simulink model "dspmrf_nbpf"  (Simulink 5.0)
settings: Solver=FixedStepDiscrete  SolverMode=SingleTasking  StartTime=0.0  StopTime=inf  RelTol=1e-3  AbsTol=1e-6
PreLoadFcn:
  | load dspmrf_coeffs
libraries: dspmlti3 x4, dspsrcs4 x2, dspsnks4 x2, dspmrf_lib x1
settings Model: Creator=don  LastModifiedBy=schim  ExtModeTrigMode=oneshot  ExtModeArmWhenConnect=off  SaveTime=off  SaveOutput=off  LimitDataPoints=off  IntegerOverflowMsg=none  BlockReductionOpt=off  BooleanDataType=off  RTWOptions=-aRollThreshold=2

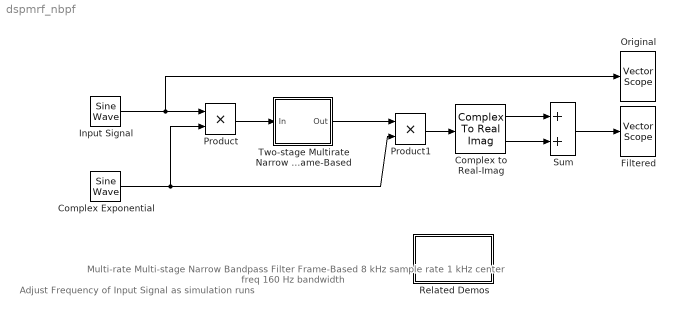
== system dspmrf_nbpf ==
  note: Multi-rate Multi-stage
      | Narrow Bandpass Filter
      | Frame-Based
      |
      | 8 kHz sample rate
      | 1 kHz center freq
      | 160 Hz bandwidth
  note: Adjust Frequency
      | of Input Signal
      | as simulation runs
  Complex Exponential : dspsrcs4/Sine Wave  Amplitude=sqrt(2)  Frequency=1000  Phase=0  SampleMode=Discrete  OutComplex=Complex  CompMethod=Table lookup  TableSize=Speed  SampleTime=1/8000  SamplesPerFrame=48  dataType=double  wordLen=16  udDataType=sfix(16)  fracBitsMode=Best precision  numFracBits=14  ResetState=Restart at time zero
  Complex to Real-Imag : ComplexToRealImag
  Filtered : dspsnks4/Vector Scope  ScopeProperties=on  Domain=Time  HorizSpan=10  DisplayProperties=off  AxisGrid=on  Memory=off  FrameNumber=off  AxisLegend=off  AxisZoom=off  OpenScopeAtSimStart=on  OpenScopeImmediately=off  FigPos=[374 163 348 280]  AxisProperties=off  XUnits=Hertz  XRange=[0...Fs/2]  InheritXIncr=on  XIncr=1  XLabel=Samples  YUnits=dB  YLabel=Amplitude  LineProperties=off  LineColors=|[1 0 0]
      settings: YMin=-1.1025  YMax=1.1025
  Input Signal : dspsrcs4/Sine Wave  Amplitude=1  Frequency=1000-40  Phase=0  SampleMode=Discrete  OutComplex=Real  CompMethod=Trigonometric fcn  TableSize=Speed  SampleTime=1/8000  SamplesPerFrame=48  dataType=double  wordLen=16  udDataType=sfix(16)  fracBitsMode=Best precision  numFracBits=14  ResetState=Restart at time zero
  Original : dspsnks4/Vector Scope  ScopeProperties=on  Domain=Time  HorizSpan=10  DisplayProperties=off  AxisGrid=on  Memory=off  FrameNumber=off  AxisLegend=off  AxisZoom=off  OpenScopeAtSimStart=on  OpenScopeImmediately=off  FigPos=[58 163 303 280]  AxisProperties=off  XUnits=Hertz  XRange=[0...Fs/2]  InheritXIncr=on  XIncr=1  XLabel=Samples  YUnits=dB  YLabel=Amplitude  LineProperties=off  LineColors=|[1 0 0]
      settings: YMin=-1.1025  YMax=1.1025
  Product : Product  SaturateOnIntegerOverflow=on  InputSameDT=on
  Product1 : Product  SaturateOnIntegerOverflow=on  InputSameDT=on
  Related Demos : Subsystem
      settings: OpenFcn=dspmrf_menu
      mask Display: disp('Other\nMultirate Filter\nDemos')
  Sum : Sum  SaturateOnIntegerOverflow=on  InputSameDT=on
  Two-stage Multirate Narrow Lowpass Frame-Based : Subsystem
  wires:
  Product/1 -> Two-stage Multirate Narrow Lowpass Frame-Based/1(In)
  Two-stage Multirate Narrow Lowpass Frame-Based/1(Out) -> Product1/1
  Product1/1 -> Complex to Real-Imag/1
  Complex to Real-Imag/1 -> Sum/1
  Complex to Real-Imag/2 -> Sum/2
  Input Signal/1 -> Product/1, Original/1
  Sum/1 -> Filtered/1
  Complex Exponential/1 -> Product/2, Product1/2

== system dspmrf_nbpf/Related Demos ==

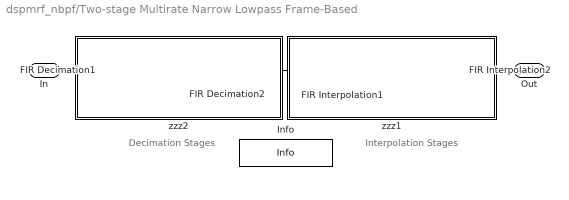
== system dspmrf_nbpf/Two-stage Multirate Narrow Lowpass Frame-Based ==
  note: Interpolation Stages
  note: Decimation Stages
  In : Inport
  FIR Decimation1 : dspmlti3/FIR Decimation  h=mrf_firdn1  D=12  framing=Maintain input frame rate
  FIR Decimation2 : dspmlti3/FIR Decimation  h=mrf_firdn2  D=4  framing=Maintain input frame rate
  FIR Interpolation1 : dspmlti3/FIR Interpolation  h=mrf_upfir2  L=4  framing=Maintain input frame rate
  FIR Interpolation2 : dspmlti3/FIR Interpolation  h=mrf_upfir1  L=12  framing=Maintain input frame rate
  Info : dspmrf_lib/Info
  zzz1 : Subsystem
      settings: OpenFcn=dspmsmrff;
      mask Display: disp('')
  zzz2 : Subsystem
      settings: OpenFcn=dspmsmrff;
      mask Display: disp('')
  Out : Outport
  wires:
  In/1 -> FIR Decimation1/1
  FIR Decimation1/1 -> FIR Decimation2/1
  FIR Decimation2/1 -> FIR Interpolation1/1
  FIR Interpolation1/1 -> FIR Interpolation2/1
  FIR Interpolation2/1 -> Out/1

== system dspmrf_nbpf/Two-stage Multirate Narrow Lowpass Frame-Based/zzz1 ==

== system dspmrf_nbpf/Two-stage Multirate Narrow Lowpass Frame-Based/zzz2 ==
